simulink model "Tyre_Pac96"  (R2023b)
settings: Solver=ode4  StartTime=0.0  StopTime=Time_sim  FixedStep=0.001  RelTol=1e-3
values from neighbouring files (symbols this model uses):
  accel_time = 0.001    [Tests.m]
  Af = 2.36    [Tests.m]
  alfa0 = 0    [Plot_Pac_Tyre_Model.m]    (also in Tests.m)
  alfa_slope = 0    [Plot_Pac_Tyre_Model.m]    (also in Tests.m)
  brake_delay = 0.02    [Tests.m]
  brake_risetime = 0.025    [Tests.m]
  brake_time = 2    [Tests.m]
  Cx = 0.27    [Tests.m]
  f0 = 0.009    [Tests.m]
  f2 = 6.5e-6    (= 6.5e-06)    [Tests.m]
  Fz0 = Fz_vet(cont1)    [Plot_Pac_Tyre_Model.m]    (also in Tests.m = 17775.72)
  Fz_slope = 0    [Plot_Pac_Tyre_Model.m]    (also in Tests.m)
  Fzr_ratio = 0.5    [Tests.m]
  gamma0 = -20    [Plot_Pac_Tyre_Model.m]    (also in Tests.m = 0)
  gamma_slope = 4    [Plot_Pac_Tyre_Model.m]    (also in Tests.m = 0)
  gear_ratio = 10.5    [Tests.m]
  inverter_eff = 0.9    [Tests.m]
  Ir = 0.675    [Tests.m]
  m = 1812    [Tests.m]
  motor_delay = 0.02    [Tests.m]
  motor_risetime = 0.05    [Tests.m]
  mu0 = mu_vet(cont1)    [Plot_Pac_Tyre_Model.m]    (also in Tests.m = 1)
  mu_slope = 0    [Plot_Pac_Tyre_Model.m]    (also in Tests.m)
  Pacn = Pace'    [Load_Tyre_Data.m]    (also in Plot_Pac_Tyre_Model.m; Tests.m)
  rho = 1.225    [Tests.m]
  s0 = 0    [Plot_Pac_Tyre_Model.m]    (also in Tests.m = 0.1)
  s_slope = 0    [Plot_Pac_Tyre_Model.m]    (also in Tests.m)
  tau_alfa = 0.1    [Tests.m]
  tau_slip = 0.1    [Tests.m]
  Tb0 = 500    [Tests.m]
  Tm0 = 2100    [Tests.m]
  transm_eff = 0.95    [Tests.m]
  V = 100/3.6    (= 27.7777777778)    [Tests.m]
  V0 = 0.1    [Tests.m]
  w0 = 0.1    [Tests.m]
  wheel_radius = 0.3    [Tests.m]
undefined symbols (not defined in the file or in its folder): Fzf_ratio
libraries: simulink x5, simulink_extras x2
settings Model: Creator=Nico  LastModifiedBy=matteo
settings SolverCC: AlgebraicLoopSolver=TrustRegion
settings DataIOCC: LimitDataPoints=on  SaveFormat=Array  SignalLoggingSaveFormat=ModelDataLogs  ReturnWorkspaceOutputs=off  SignalLoggingName=sigsOut
settings OptimizationCC: BooleanDataType=off  InitFltsAndDblsToZero=on  LifeSpan=inf
settings DebuggingCC: SaveWithParameterizedLinksMsg=none  UnderspecifiedInitializationDetection=Classic  MergeDetectMultiDrivingBlocksExec=none  SignalResolutionControl=TryResolveAllWithWarning  MultiTaskDSMMsg=warning  MultiTaskCondExecSysMsg=none  FcnCallInpInsideContextMsg=warning  UnconnectedInputMsg=warning  UnconnectedOutputMsg=warning  UnconnectedLineMsg=warning  AllowSymbolicDim=off  SFUnexpectedBacktrackingDiag=warning  SFNoUnconditionalDefaultTransitionDiag=warning  SFExecutionAtInitializationDiag=none  ArithmeticOperatorsInVariantConditions=warning
settings HardwareCC: ProdBitPerPointer=32  ProdBitPerSizeT=32  ProdBitPerPtrDiffT=32  ProdLargestAtomicFloat=None  ProdIntDivRoundTo=Undefined  ProdEndianess=Unspecified  ProdWordSize=32  ProdHWDeviceType=32-bit Generic  TargetUnknown=on
settings ModelReferenceCC: EnableRefExpFcnMdlSchedulingChecks=on  PropagateSignalLabelsOutOfModel=off
settings SFSimCC: SimUseLocalCustomCode=off  SimParseCustomCode=off  CustomCodeUndefinedFunction=UseInterfaceOnly
settings RTWCC: RTWUseLocalCustomCode=off  DLArmComputeVersion=19.05
settings CodeAppCC: StateflowObjectComments=on
settings GRTTargetCC: TargetFcnLib=ansi_tfl_tmw.mat  TargetLangStandard=C89/C90 (ANSI)  CombineOutputUpdateFcns=off  GRTInterface=on
settings ConfigComp: CovMetricSettings=dw  CovSaveCumulativeToWorkspaceVar=on  CovSaveSingleToWorkspaceVar=on  CovExternalEMLEnable=off

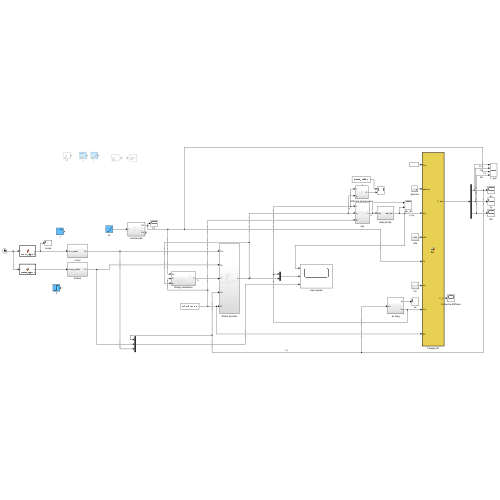
[thumbnail: Simulink's stored preview of the top-level diagram]
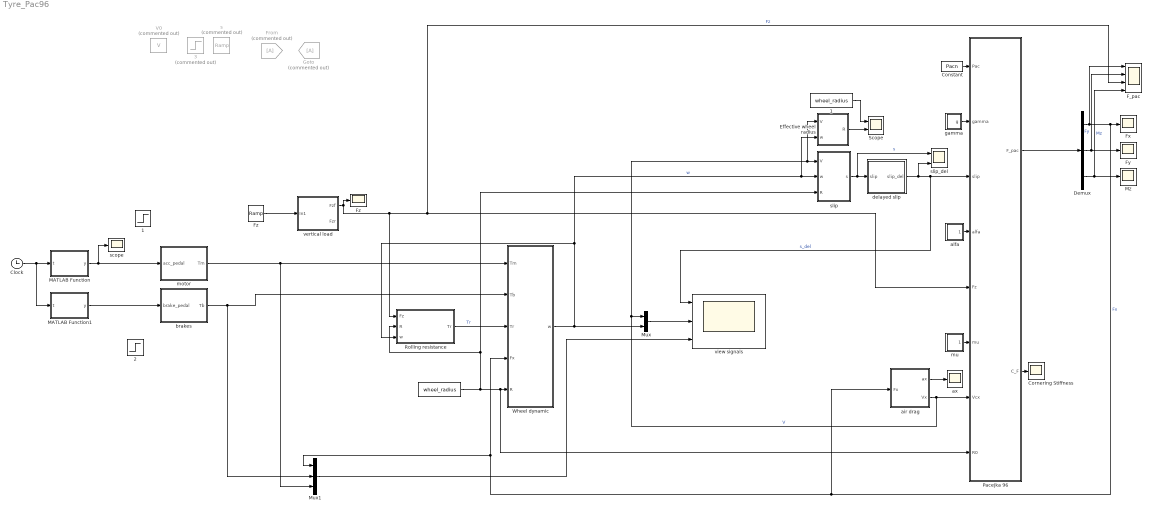
== system Tyre_Pac96 ==
  "   " : Constant  Value=wheel_radius
  "   1" : Constant  Value=wheel_radius
  " 1" : Step  Time=accel_time  After=Tm0  SampleTime=0
  " 2" : Step  Time=brake_time  After=Tb0  SampleTime=0
  " 3" : Step  Commented=on  Before=1  After=0.1  SampleTime=0
  Clock : Clock
  Constant : Constant  Value=Pacn
  Cornering Stiffness : Scope
  Demux : Demux  Outputs=3
  Effective wheel radius : Subsystem
  F_pac : Scope  NumInputPorts=4
  From : From  Commented=on
  Fx : Scope
  Fy : Scope
  Fz : simulink/Sources/Ramp  slope=Fz_slope  start=1  InitialOutput=Fz0
  "Fz " : Scope
  Goto : Goto  Commented=on
  MATLAB Function : MATLAB Function  TreatAsAtomicUnit=on
  MATLAB Function1 : MATLAB Function  TreatAsAtomicUnit=on
  Mux : Mux  Inputs=2
  Mux1 : Mux  Inputs=3
  Mz : Scope
  Pacejka 96 : MATLAB Function  TreatAsAtomicUnit=on
  Rolling resistance : Subsystem
  Scope : Scope  NumInputPorts=2
  V0 : Constant  Commented=on  Value=V
  Wheel dynamic : Subsystem
  air drag : Subsystem
  alfa : Subsystem
  ax : Scope
  brakes : Subsystem
  delayed slip : Subsystem
  gamma : Subsystem
  motor : Subsystem
  mu : Subsystem
  "s " : simulink/Sources/Ramp  Commented=on  slope=s_slope  start=1  InitialOutput=s0
  scope : Scope
  slip : Subsystem
  slip_del : Scope  NumInputPorts=2
  vertical load : Subsystem
  view signals : Scope  NumInputPorts=3
  wires:
  Constant/1 -> Pacejka 96/1(Pac)
  Pacejka 96/1(F_pac) -> Demux/1
  Pacejka 96/2(C_F) -> Cornering Stiffness/1
  Demux/1 -> F_pac/1, Wheel dynamic/4(Fx), Mux1/1, air drag/1(Fx), Fx/1  "Fx"
  Demux/2 -> F_pac/2, Fy/1  "Fy"
  Demux/3 -> F_pac/4, Mz/1  "Mz"
  vertical load/1(Fzf) -> Pacejka 96/5(Fz), F_pac/3, Rolling resistance/1(Fz), "Fz "/1  "Fz"
  air drag/1(ax) -> ax/1
  "   "/1 -> Wheel dynamic/5(R), Pacejka 96/8(R0), Rolling resistance/2(R), slip/3(R)
  Rolling resistance/1(Tr) -> Wheel dynamic/3(Tr)  "Tr"
  Wheel dynamic/1(w) -> Effective wheel radius/2(w), slip/2(w), Rolling resistance/3(w), Mux/2  "w"
  motor/1(Tm) -> Mux1/3, Wheel dynamic/1(Tm)
  brakes/1(Tb) -> Mux1/2, Wheel dynamic/2(Tb)
  air drag/2(Vx) -> Pacejka 96/7(Vcx), Effective wheel radius/1(V), slip/1(V), Mux/1  "V"
  Fz/1 -> vertical load/1(In1)
  slip/1(s) -> slip_del/1, delayed slip/1(slip)  "s"
  alfa/1("alfa  ") -> Pacejka 96/4(alfa)
  gamma/1(g) -> Pacejka 96/2(gamma)
  Mux/1 -> view signals/2
  Mux1/1 -> view signals/3
  delayed slip/1(slip_del) -> slip_del/2, Pacejka 96/3(slip), view signals/1  "s_del"
  mu/1(Out1) -> Pacejka 96/6(mu)
  Clock/1 -> MATLAB Function1/1(t), MATLAB Function/1(t)
  MATLAB Function/1(y) -> motor/1(acc_pedal), scope/1
  MATLAB Function1/1(y) -> brakes/1(brake_pedal)
  Effective wheel radius/1(R) -> Scope/2
  "   1"/1 -> Scope/1

== system Tyre_Pac96/Effective wheel radius ==
  V : Inport
  w : Inport  Port=2
  Divide : Product  Inputs=*/
  R : Outport
  wires:
  V/1 -> Divide/1
  w/1 -> Divide/2
  Divide/1 -> R/1

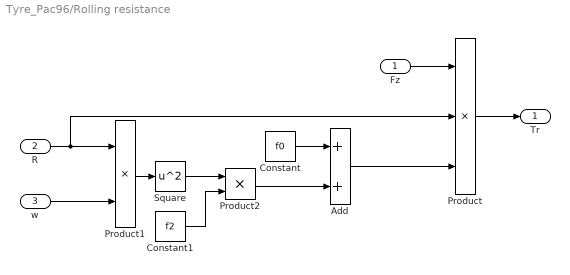
== system Tyre_Pac96/Rolling resistance ==
  Fz : Inport
  R : Inport  Port=2
  w : Inport  Port=3
  Add : Sum
  Constant : Constant  Value=f0
  Constant1 : Constant  Value=f2
  Product : Product  Inputs=3
  Product1 : Product
  Product2 : Product
  Square : Math  Operator=square
  Tr : Outport
  wires:
  Fz/1 -> Product/1
  w/1 -> Product1/2
  Constant/1 -> Add/1
  R/1 -> Product/2, Product1/1
  Product1/1 -> Square/1
  Square/1 -> Product2/1
  Constant1/1 -> Product2/2
  Product2/1 -> Add/2
  Add/1 -> Product/3
  Product/1 -> Tr/1

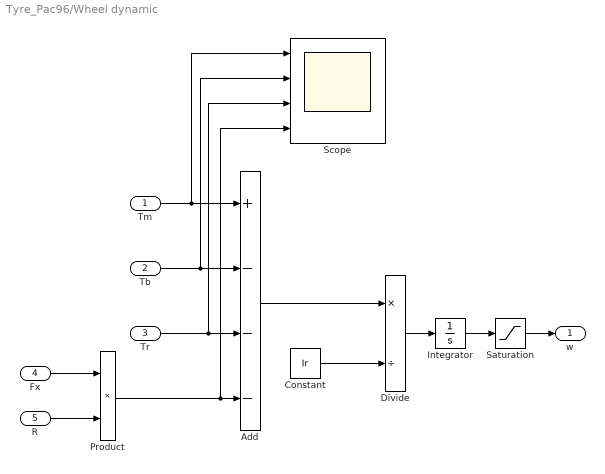
== system Tyre_Pac96/Wheel dynamic ==
  Tm : Inport
  Tb : Inport  Port=2
  Tr : Inport  Port=3
  Fx : Inport  Port=4
  R : Inport  Port=5
  Add : Sum  Inputs=+---
  Constant : Constant  Value=Ir
  Divide : Product  Inputs=*/
  Integrator : Integrator  InitialCondition=w0
  Product : Product
  Saturation : Saturate  UpperLimit=1e20  LowerLimit=0.00000001
  Scope : Scope  NumInputPorts=4
  w : Outport
  wires:
  Fx/1 -> Product/1
  R/1 -> Product/2
  Tm/1 -> Scope/1, Add/1
  Tb/1 -> Scope/2, Add/2
  Product/1 -> Add/4, Scope/4
  Add/1 -> Divide/1
  Constant/1 -> Divide/2
  Divide/1 -> Integrator/1
  Integrator/1 -> Saturation/1
  Tr/1 -> Scope/3, Add/3
  Saturation/1 -> w/1

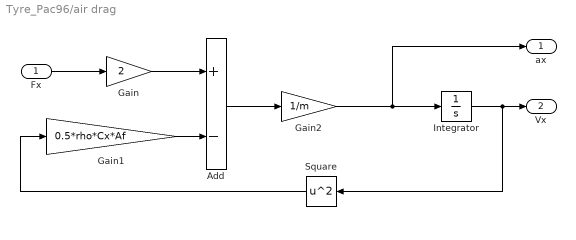
== system Tyre_Pac96/air drag ==
  Fx : Inport
  Add : Sum  Inputs=+-
  Gain : Gain  Gain=2
  Gain1 : Gain  Gain=0.5*rho*Cx*Af
  Gain2 : Gain  Gain=1/m
  Integrator : Integrator  InitialCondition=V0
  Square : Math  Operator=square
  ax : Outport
  Vx : Outport  Port=2
  wires:
  Fx/1 -> Gain/1
  Gain/1 -> Add/1
  Gain1/1 -> Add/2
  Square/1 -> Gain1/1
  Add/1 -> Gain2/1
  Gain2/1 -> ax/1, Integrator/1
  Integrator/1 -> Square/1, Vx/1

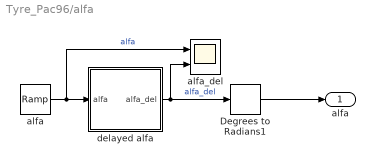
== system Tyre_Pac96/alfa ==
  Degrees to Radians1 : simulink_extras/Transformations/Degrees to Radians
  alfa : simulink/Sources/Ramp  slope=alfa_slope  start=1  InitialOutput=alfa0
  alfa_del : Scope  NumInputPorts=2
  delayed alfa : Subsystem
  "alfa  " : Outport
  wires:
  alfa/1 -> alfa_del/1, delayed alfa/1(alfa)  "alfa"
  delayed alfa/1(alfa_del) -> Degrees to Radians1/1, alfa_del/2  "alfa_del"
  Degrees to Radians1/1 -> "alfa  "/1

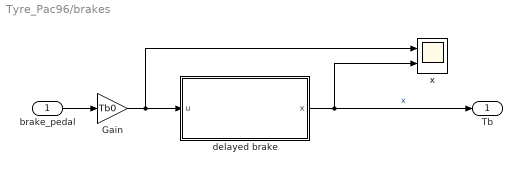
== system Tyre_Pac96/brakes ==
  brake_pedal : Inport
  Gain : Gain  Gain=Tb0
  delayed brake : Subsystem
  x : Scope  NumInputPorts=2
  Tb : Outport
  wires:
  brake_pedal/1 -> Gain/1
  delayed brake/1(x) -> Tb/1, x/2  "x"
  Gain/1 -> x/1, delayed brake/1(u)

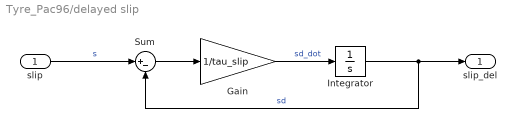
== system Tyre_Pac96/delayed slip ==
  slip : Inport
  Gain : Gain  Gain=1/tau_slip
  Integrator : Integrator  InitialCondition=s0
  Sum : Sum  Inputs=|+-
  slip_del : Outport
  wires:
  slip/1 -> Sum/1  "s"
  Integrator/1 -> Sum/2, slip_del/1  "sd"
  Gain/1 -> Integrator/1  "sd_dot"
  Sum/1 -> Gain/1

== system Tyre_Pac96/gamma ==
  Degrees to Radians : simulink_extras/Transformations/Degrees to Radians
  gamma : simulink/Sources/Ramp  slope=gamma_slope  start=1  InitialOutput=gamma0
  "gamma " : Scope
  g : Outport
  wires:
  gamma/1 -> "gamma "/1, Degrees to Radians/1
  Degrees to Radians/1 -> g/1

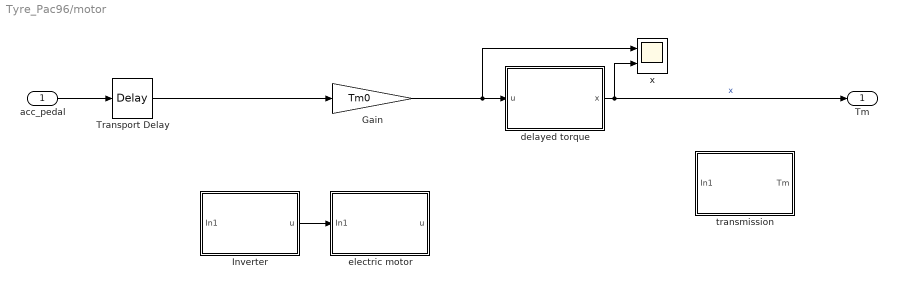
== system Tyre_Pac96/motor ==
  acc_pedal : Inport
  Gain : Gain  Gain=Tm0
  Inverter : Subsystem
  Transport Delay : TransportDelay  DelayTime=motor_delay
  delayed torque : Subsystem
  electric motor : Subsystem
  transmission : Subsystem
  x : Scope  NumInputPorts=2
  Tm : Outport
  wires:
  delayed torque/1(x) -> Tm/1, x/2  "x"
  Inverter/1(u) -> electric motor/1(In1)
  acc_pedal/1 -> Transport Delay/1
  Transport Delay/1 -> Gain/1
  Gain/1 -> x/1, delayed torque/1(u)

== system Tyre_Pac96/mu ==
  mu : simulink/Sources/Ramp  slope=mu_slope  start=1  InitialOutput=mu0
  "mu " : Scope
  Out1 : Outport
  wires:
  mu/1 -> Out1/1, "mu "/1

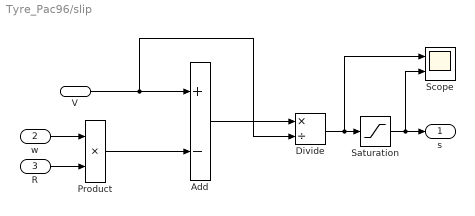
== system Tyre_Pac96/slip ==
  V : Inport
  w : Inport  Port=2
  R : Inport  Port=3
  Add : Sum  Inputs=+-
  Divide : Product  Inputs=*/
  Product : Product
  Saturation : Saturate  UpperLimit=1  LowerLimit=-1e100
  Scope : Scope  NumInputPorts=2
  s : Outport
  wires:
  V/1 -> Divide/2, Add/1
  Add/1 -> Divide/1
  w/1 -> Product/1
  R/1 -> Product/2
  Product/1 -> Add/2
  Divide/1 -> Scope/1, Saturation/1
  Saturation/1 -> Scope/2, s/1

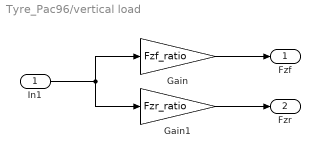
== system Tyre_Pac96/vertical load ==
  In1 : Inport
  Gain : Gain  Gain=Fzf_ratio
  Gain1 : Gain  Gain=Fzr_ratio
  Fzf : Outport
  Fzr : Outport  Port=2
  wires:
  In1/1 -> Gain/1, Gain1/1
  Gain/1 -> Fzf/1
  Gain1/1 -> Fzr/1

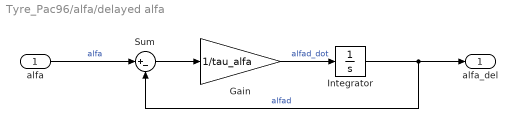
== system Tyre_Pac96/alfa/delayed alfa ==
  alfa : Inport
  Gain : Gain  Gain=1/tau_alfa
  Integrator : Integrator  InitialCondition=alfa0
  Sum : Sum  Inputs=|+-
  alfa_del : Outport
  wires:
  Sum/1 -> Gain/1
  Gain/1 -> Integrator/1  "alfad_dot"
  Integrator/1 -> alfa_del/1, Sum/2  "alfad"
  alfa/1 -> Sum/1  "alfa"

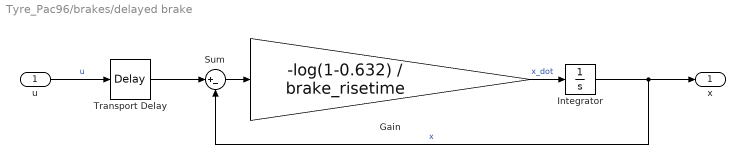
== system Tyre_Pac96/brakes/delayed brake ==
  u : Inport
  Gain : Gain  Gain=-log(1-0.632) / brake_risetime
  Integrator : Integrator
  Sum : Sum  Inputs=|+-
  Transport Delay : TransportDelay  DelayTime=brake_delay
  x : Outport
  wires:
  Sum/1 -> Gain/1
  Gain/1 -> Integrator/1  "x_dot"
  Integrator/1 -> x/1, Sum/2  "x"
  u/1 -> Transport Delay/1  "u"
  Transport Delay/1 -> Sum/1

== system Tyre_Pac96/motor/Inverter ==
  In1 : Inport
  Gain : Gain  Gain=inverter_eff
  u : Outport
  wires:
  In1/1 -> Gain/1
  Gain/1 -> u/1

== system Tyre_Pac96/motor/delayed torque ==
  u : Inport
  Gain : Gain  Gain=-log(1-0.632) / motor_risetime
  Integrator : Integrator
  Sum : Sum  Inputs=|+-
  x : Outport
  wires:
  Sum/1 -> Gain/1
  Gain/1 -> Integrator/1  "x_dot"
  Integrator/1 -> x/1, Sum/2  "x"
  u/1 -> Sum/1  "u"

== system Tyre_Pac96/motor/electric motor ==
  In1 : Inport
  Gain : Gain  Gain=Tm0
  u : Outport
  wires:
  In1/1 -> Gain/1
  Gain/1 -> u/1

== system Tyre_Pac96/motor/transmission ==
  note: 2 wheels
  In1 : Inport
  Gain1 : Gain  Gain=transm_eff
  Gain2 : Gain  Gain=1/gear_ratio
  Gain3 : Gain  Gain=0.5
  Tm : Outport
  wires:
  In1/1 -> Gain2/1
  Gain1/1 -> Gain3/1
  Gain2/1 -> Gain1/1
  Gain3/1 -> Tm/1

== matlab function Tyre_Pac96/Pacejka 96 ==
  settings: fimath=|
      | fimath(...
      | 'RoundMode', 'floor',...
      | 'OverflowMode', 'wrap',...
      | 'ProductMode', 'KeepLSB', 'ProductWordLength', 32,...
      | 'SumMode', 'KeepLSB', 'SumWordLength', 32,...
      | 'CastBeforeSum', false)
  data: Pac input; gamma input; slip input; alfa input; Fz input; F_pac output; mu input; Vcx input; C_F output; R0 input
function [F_pac,C_F] = fcn(Pac,gamma,slip,alfa,Fz,mu,Vcx,R0)
% function for computing forces Fx, Fy and self-aligning torque Mz

% Pac   -> model structure with coeff. Pacejka 96
% slip  -> slip ratio [-] (-1:1)
% alfa  -> slip angle [rad]
% gamma -> camber [rad]
% Vcx,y velocity components of tire contact point C

% Structure building: Pacejka model coefficients
Pa_FZ0_ = Pac(1);
Pa_LFZ0 = Pac(2);
Pa_LmuV = Pac(3);
Pa_LKXK = Pac(4);
Pa_LKYA = Pac(5);
Pa_LCX_ = Pac(6);
Pa_LCY_ = Pac(7);
Pa_LEX_ = Pac(8);
Pa_LEY_ = Pac(9);
Pa_LHX_ = Pac(10);
Pa_LHY_ = Pac(11);
Pa_LVX_ = Pac(12);
Pa_LVY_ = Pac(13);
Pa_LKYG = Pac(14);
Pa_LKZG = Pac(15);
Pa_LT__ = Pac(16);
Pa_MR__ = Pac(17);
Pa_LXA_ = Pac(18);
Pa_LYK_ = Pac(19);
Pa_LVYK = Pac(20);
Pa_LS__ = Pac(21);
Pa_LCZ_ = Pac(22);
Pa_LMX_ = Pac(23);
Pa_LMY_ = Pac(24);
Pa_PCX1 = Pac(25);
Pa_PDX1 = Pac(26);
Pa_PDX2 = Pac(27);
Pa_PEX1 = Pac(28);
Pa_PEX2 = Pac(29);
Pa_PEX3 = Pac(30);
Pa_PEX4 = Pac(31);
Pa_PKX1 = Pac(32);
Pa_PKX2 = Pac(33);
Pa_PKX3 = Pac(34);
Pa_PHX1 = Pac(35);
Pa_PHX2 = Pac(36);
Pa_PVX1 = Pac(37);
Pa_PVX2 = Pac(38);
Pa_RBX1 = Pac(39);
Pa_RBX2 = Pac(40);
Pa_RCX1 = Pac(41);
Pa_RHX1 = Pac(42);
Pa_RTX1 = Pac(43);
Pa_RTX2 = Pac(44);
Pa_RTX3 = Pac(45);
Pa_QSX1 = Pac(46);
Pa_QSX2 = Pac(47);
Pa_QSX3 = Pac(48);
Pa_PCY1 = Pac(49);
Pa_PDY1 = Pac(50);
Pa_PDY2 = Pac(51);
Pa_PDY3 = Pac(52);
Pa_PEY1 = Pac(53);
Pa_PEY2 = Pac(54);
Pa_PEY3 = Pac(55);
Pa_PEY4 = Pac(56);
Pa_PKY1 = Pac(57);
Pa_PKY2 = Pac(58);
Pa_PKY3 = Pac(59);
Pa_PHY1 = Pac(60);
Pa_PHY2 = Pac(61);
Pa_PHY3 = Pac(62);
Pa_PVY1 = Pac(63);
Pa_PVY2 = Pac(64);
Pa_PVY3 = Pac(65);
Pa_PVY4 = Pac(66);
Pa_RBY1 = Pac(67);
Pa_RBY2 = Pac(68);
Pa_RBY3 = Pac(69);
Pa_RCY1 = Pac(70);
Pa_RHY1 = Pac(71);
Pa_RVY1 = Pac(72);
Pa_RVY2 = Pac(73);
Pa_RVY3 = Pac(74);
Pa_RVY4 = Pac(75);
Pa_RVY5 = Pac(76);
Pa_RVY6 = Pac(77);
Pa_PTY1 = Pac(78);
Pa_PTY2 = Pac(79);
Pa_QSY1 = Pac(80);
Pa_QSY2 = Pac(81);
Pa_QBZ1 = Pac(82);
Pa_QBZ2 = Pac(83);
Pa_QBZ3 = Pac(84);
Pa_QBZ4 = Pac(85);
Pa_QBZ5 = Pac(86);
Pa_QBZ6 = Pac(87);
Pa_QBZ9 = Pac(88);
Pa_QBZZ = Pac(89);
Pa_QCZ1 = Pac(90);
Pa_QDZ1 = Pac(91);
Pa_QDZ2 = Pac(92);
Pa_QDZ3 = Pac(93);
Pa_QDZ4 = Pac(94);
Pa_QDZ6 = Pac(95);
Pa_QDZ7 = Pac(96);
Pa_QDZ8 = Pac(97);
Pa_QDZ9 = Pac(98);
Pa_QEZ1 = Pac(99);
Pa_QEZ2 = Pac(100);
Pa_QEZ3 = Pac(101);
Pa_QEZ4 = Pac(102);
Pa_QEZ5 = Pac(103);
Pa_QHZ1 = Pac(104);
Pa_QHZ2 = Pac(105);
Pa_QHZ3 = Pac(106);
Pa_QHZ4 = Pac(107);
Pa_SSZ1 = Pac(108);
Pa_SSZ2 = Pac(109);
Pa_SSZ3 = Pac(110);
Pa_SSZ4 = Pac(111);
Pa_QTZ1 = Pac(112);

% Costants
epsi = 0.01;
eps_V = 0.1;
csi_0=1;
csi_4=1;
Amu = 10;
Pa_LmuX = mu;
Pa_LmuY = mu;

%-------------------------------- Fx pure slip ---------------------------
Cx = Pa_PCX1*Pa_LCX_;
dfz = (Fz-Pa_LFZ0*Pa_FZ0_)/(Pa_LFZ0*Pa_FZ0_);
mux = Pa_LmuX * (Pa_PDX1 + Pa_PDX2 * dfz);
Dx = mux*Fz; %*csi_1, con csi_1=1
%Shx = (Pa_PHX1+Pa_PHX2*dfz)*Pa_LHX_;
Shx = 0;
Kx = slip + Shx;
Ex = (Pa_PEX1+Pa_PEX2*dfz+Pa_PEX3*dfz^2)*(1-Pa_PEX4*sign(Kx))*Pa_LEX_;
if Ex>1 Et=1; end
Kxk = Fz*(Pa_PKX1+Pa_PKX2*dfz)*exp(Pa_PKX3*dfz)*Pa_LKXK;
Bx = Kxk/(Cx*Dx+epsi);
lam_mux  = Pa_LmuX*Amu/(1+(Amu-1)*Pa_LmuX);
SVx = Fz*(Pa_PVX1+Pa_PVX2*dfz)*(abs(Vcx)/(abs(Vcx)+eps_V))*Pa_LVX_*lam_mux; %*csi_1, con csi_1=1

% logitudinal slip stiffness (Fx slope in the origin)
C_Fk = Bx*Cx*Dx;

% longitudinal force
Fx0 = Dx*sin(Cx*atan(Bx*Kx-Ex*(Bx*Kx-atan(Bx*Kx)))) + SVx;

%---------------------------- Fy pure side slip --------------------------
seg=sign(Vcx);
if seg==0 seg=1; end
alfa_star = tan(alfa)*seg;
gam_star = sin(gamma);
Shy = (Pa_PHY1+Pa_PHY2*dfz)*Pa_LHY_+Pa_PHY3*gam_star*Pa_LKYG*csi_0+csi_4-1;
alfa_y = alfa_star + Shy;
Cy = Pa_PCY1*Pa_LCY_;
muy = Pa_LmuY*(Pa_PDY1+Pa_PDY2*dfz)*(1-Pa_PDY3*gam_star^2);
Dy = muy*Fz; %*csi_2, con csi_2=1
Ey = (Pa_PEY1+Pa_PEY2*dfz)*(1-(Pa_PEY3+Pa_PEY4*gam_star)*sign(alfa_y))*Pa_LEY_;
if Ey>1 Ey=1; end
Kya0 = Pa_PKY1*Pa_LFZ0*Pa_FZ0_*sin(2*atan(Fz/(Pa_PKY2*Pa_LFZ0*Pa_FZ0_)))*Pa_LKYA;
Kya = Kya0*(1-Pa_PKY3*gam_star^2); %*csi_3, con csi_3=1
By = Kya/(Cy*Dy+epsi);
lam_muy = Pa_LmuY*Amu/(1+(Amu-1)*Pa_LmuY);
SVy = Fz*((Pa_PVY1+Pa_PVY2*dfz)*Pa_LVY_+(Pa_PVY3+Pa_PVY4*dfz)*gam_star*Pa_LKYG )*lam_muy; %*csi_2, con csi_2=1
Kyg0 = (Pa_PHY3*Kya0+Fz*(Pa_PVY3+Pa_PVY4*dfz))*Pa_LKYG;

% cornering stiffness (Fy slope in the origin)
C_Fa = By*Cy*Dy;

% lateral force
Fy0 = Dy*sin(Cy*atan(By*alfa_y-Ey*(By*alfa_y-atan(By*alfa_y)))) + SVy;

% --------------------- Fx combined slip ------------------------------
Shxa = Pa_RHX1;
%Exa = Pa_REX1+Pa_REX2*dfz; NON esiste Pa.REX1 ne' Pa.REX2
Exa = 0;
Cxa = Pa_RCX1;
Bxa = Pa_RBX1*cos(atan(Pa_RBX2*slip))*Pa_LXA_;
alfaS = alfa_star+Shxa;
Gxa0 = cos(Cxa*atan(Bxa*Shxa-Exa*(Bxa*Shxa-atan(Bxa*Shxa))));
Gxa = cos(Cxa*atan(Bxa*alfaS-Exa*(Bxa*alfaS-atan(Bxa*alfaS))))/Gxa0;
Fx = Fx0*Gxa;

% ---------------------- Fy combined slip ------------------------------
Dvyk = muy*Fz*(Pa_RVY1+Pa_RVY2*dfz+Pa_RVY3*gam_star)*cos(atan(Pa_RVY4*alfa_star));%*csi_2, con csi_2=1
Svyk = Dvyk*sin(Pa_RVY5*atan(Pa_RVY6*slip));
Shyk = Pa_RHY1; %+Pa.RHY2*dfz; NON esiste Pa.RHY2
Cyk = Pa_RCY1;
Byk = Pa_RBY1*cos(atan(Pa_RBY2*(alfa_star-Pa_RBY3)))*Pa_LYK_;
%Eyk = Pa_REY1+Pa_REY2*dfz; NON esiste Pa.REY1 ne' Pa.REY2
Eyk = 0;
ks = slip+Shyk;
Gyk0 = cos(Cyk*atan(Byk*Shyk-Eyk*(Byk*Shyk-atan(Byk*Shyk))));
Gyk = cos(Cyk*atan(Byk*ks-Eyk*(Byk*ks-atan(Byk*ks))))/Gyk0;
Fy = Fy0*Gyk+Svyk;

% --------------------- Mz pure side slip  ---------------------------
Shf = Shy+SVy/Kya;
alfa_r = alfa_star+Shf;
Br = (Pa_QBZ9/Pa_LmuY+Pa_QBZZ*By*Cy); %*csi_6, con csi_6=1
%%% Pa_QBZZ e' in realta' QBZ10 scritto cosi' x ragioni di spazio
Cr = 1; %*csi_7, con csi_7=1
Dr = Fz*R0*((Pa_QDZ6+Pa_QDZ7*dfz)+(Pa_QDZ8+Pa_QDZ9*dfz)*gam_star)*cos(alfa)*Pa_LmuY*seg; %+csi_8-1, con csi_8=1
Mzr0 = Dr*cos(Cr*atan(Br*alfa_r));
Sht = Pa_QHZ1+Pa_QHZ2*dfz+(Pa_QHZ3+Pa_QHZ4*dfz)*gam_star;
alfa_t = alfa_star+Sht;
Bt = (Pa_QBZ1+Pa_QBZ2*dfz+Pa_QBZ3*dfz^2)*(1+Pa_QBZ5*abs(gam_star)+Pa_QBZ6*gam_star^2)*Pa_LKYA/Pa_LmuY;
if Bt<0 Bt=0; end
Ct = Pa_QCZ1;
Dt0 = Fz*R0/(Pa_LFZ0*Pa_FZ0_)*(Pa_QDZ1+Pa_QDZ2*dfz)*seg;
Dt = Dt0*(1+Pa_QDZ3*abs(gam_star)+Pa_QDZ4*gam_star^2); %*csi_5, con csi_5=1
Et = (Pa_QEZ1+Pa_QEZ2*dfz+Pa_QEZ3*dfz^2)*(1+(Pa_QEZ4+Pa_QEZ5*gam_star)*2/pi*atan(Bt*Ct*alfa_t));
if Et>1 Et=1; end
t0 = Dt*cos(Ct*atan(Bt*alfa_t - Et*(Bt*alfa_t-atan(Bt*alfa_t))))*cos(alfa);
Mz0 = -t0*Fy;
Kza0 = Dt0*Kya0;
%Kzg0 = Fz*R0*(Pa_QDZ8+Pa_QDZ9*dfz)-Dt0*Kyg0;

% aligning torque
Mz = Mz0 + Mzr0;

% ------------------------ Mz Combined -----------------------------
eps_k = 0; % 
lambda_s = Pa_LS__ ;
Fz0p = Pa_LFZ0*Pa_FZ0_;
K_yap = Kya + eps_k;
alfa_req = sqrt(alfa_r^2+(Kxk/K_yap)^2*slip^2)*sign(alfa_r);
alfa_teq = sqrt(alfa_t^2+(Kxk/K_yap)^2*slip^2)*sign(alfa_t);
s = R0*(Pa_SSZ1 + Pa_SSZ2*(Fy/Fz0p) + (Pa_SSZ3+Pa_SSZ4*dfz)*gam_star)*lambda_s;
Mzr = Dr*cos(Cr*atan(Br*alfa_req));
Fyp = Fy-Svyk; 
t = Dt*cos(Ct*atan(Bt*alfa_teq - Et*(Bt*alfa_teq-atan(Bt*alfa_teq))))*cos(alfa);
Mzp = -t*Fyp;
% aligning torque
Mz = Mzp + Mzr + s*Fx;
%%%%%%%%%%%%%%%%%%%%%%%

% Check that Fz is positive
if Fz <= 0
    Fx = 0;
    Fy = 0;
    Mz = 0;
end

% Output
F_pac = [Fx; Fy; Mz];
C_F = [C_Fk; C_Fa];

== matlab function Tyre_Pac96/MATLAB Function ==
  data: t input; y output
function y = motor_signal(t)

if t < 0.001
    y = 0;
elseif t < 7
    y = 1;
else
    y = 0;

end

== matlab function Tyre_Pac96/MATLAB Function1 ==
  data: t input; y output
function y = brake_signal(t)

if t < 7
    y = 0;
else
    y = 1;

end
